simulink model "zad6popraw"  (R2023a)
settings: Solver=VariableStepAuto  StartTime=0.0  StopTime=100  RelTol=1e-3
model workspace (MAT data in the model file):
  T = Simulink.Parameter
  T.Value = 3
  T.DataType = 'auto'
  T.Complexity = 'real'
  T.Dimensions = [1 1]
  T1 = Simulink.Parameter
  T1.Value = 9
  T1.DataType = 'auto'
  T1.Complexity = 'real'
  T1.Dimensions = [1 1]
  T2 = Simulink.Parameter
  T2.Value = 8
  T2.DataType = 'auto'
  T2.Complexity = 'real'
  T2.Dimensions = [1 1]
values from neighbouring files (symbols this model uses):
  a1 = -0.8    [zad10.m]    (also in zad2.m; zad3.m)
  a2 = -0.86    [zad10.m]    (also in zad2.m; zad3.m)
  a3 = -0.41    [zad10.m]    (also in zad2.m; zad3.m)
  a4 = -0.41    [zad10.m]    (also in zad2.m; zad3.m)
  K = 1    [zad10.m]    (also in zad2.m; zad3.m)
  T = 1    [zad10.m]
  T1 = 9    [zad10.m]
  T2 = 8    [zad10.m]
settings Model: Creator=pkutyl  LastModifiedBy=pkutyl

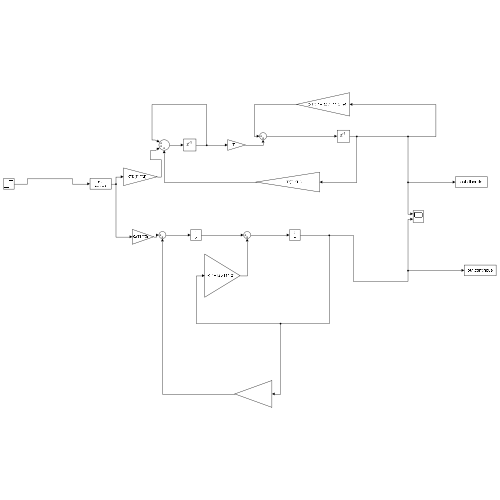
[thumbnail: Simulink's stored preview of the top-level diagram]
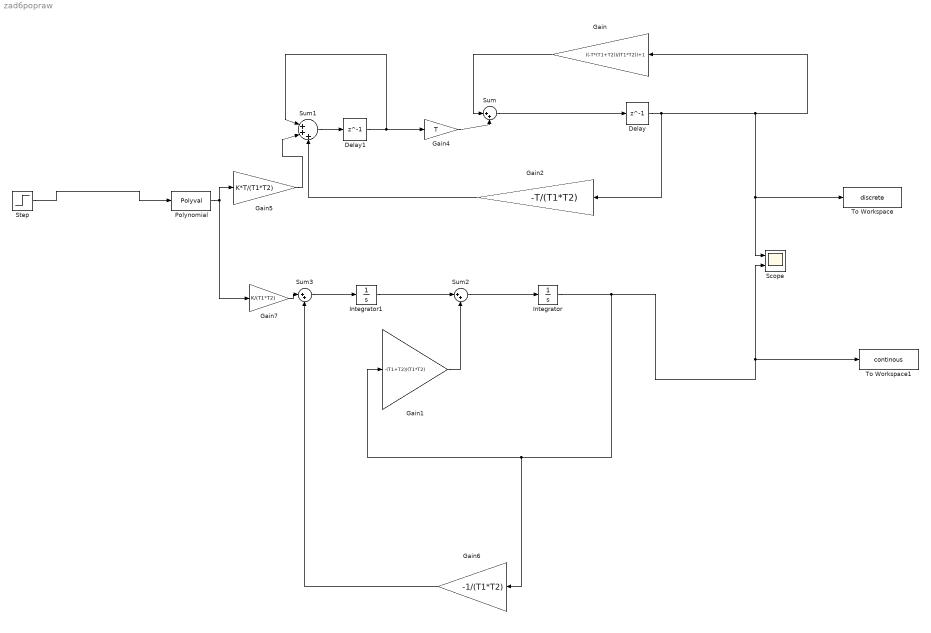
== system zad6popraw ==
  Delay : Delay  DelayLength=1  InitialCondition=0  SampleTime=T
  Delay1 : Delay  DelayLength=1  InitialCondition=0  SampleTime=T
  Gain : Gain  Gain=((-T*(T1+T2))/(T1*T2))+1
  Gain1 : Gain  Gain=-(T1+T2)/(T1*T2)
  Gain2 : Gain  Gain=-T/(T1*T2)
  Gain4 : Gain  Gain=T
  Gain5 : Gain  Gain=K*T/(T1*T2)
  Gain6 : Gain  Gain=-1/(T1*T2)
  Gain7 : Gain  Gain=K/(T1*T2)
  Integrator : Integrator
  Integrator1 : Integrator
  Polynomial : Polyval  Coefs=[a4,a3,a2,a1,0]
  Scope : Scope  NumInputPorts=2
  Step : Step  SampleTime=0
  Sum : Sum  Inputs=|++
  Sum1 : Sum  Inputs=|+++
  Sum2 : Sum  Inputs=|++
  Sum3 : Sum  Inputs=|++
  To Workspace : ToWorkspace  VariableName=discrete  SaveFormat=Structure With Time  SampleTime=-1
  To Workspace1 : ToWorkspace  VariableName=continous  SaveFormat=Structure With Time  SampleTime=-1
  wires:
  Gain5/1 -> Sum1/2
  Gain4/1 -> Sum/2
  Sum/1 -> Delay/1
  Delay/1 -> Gain2/1, To Workspace/1, Scope/1, Gain/1
  Gain/1 -> Sum/1
  Delay1/1 -> Sum1/1, Gain4/1
  Gain2/1 -> Sum1/3
  Sum1/1 -> Delay1/1
  Step/1 -> Polynomial/1
  Gain1/1 -> Sum2/2
  Gain7/1 -> Sum3/1
  Sum2/1 -> Integrator/1
  Polynomial/1 -> Gain7/1, Gain5/1
  Gain6/1 -> Sum3/2
  Sum3/1 -> Integrator1/1
  Integrator1/1 -> Sum2/1
  Integrator/1 -> Scope/2, To Workspace1/1, Gain1/1, Gain6/1
